simulink model "banc_essai_dec"  (R2021a)
settings: Solver=ode45  StartTime=0.0  StopTime=tfin  FixedStep=0.001  RelTol=1e-09  EnableMultiTasking=on
values from neighbouring files (symbols this model uses):
  A_phi = [A_plaque(1,1),    A_plaque(1,4),  A_plaque(1,7) ... (first row only)    [decouplage.m]
  A_teta = [A_plaque(2,2),    A_plaque(2,5),  A_plaque(2,8) ... (first row only)    [decouplage.m]
  A_x = [A_sphere(1,1), A_sphere(1,3) ... (first row only)    [decouplage.m]
  A_y = [A_sphere(2,2), A_sphere(2,4) ... (first row only)    [decouplage.m]
  A_z = [A_plaque(3,3),    A_plaque(3,6),  A_plaque(3,9) ... (first row only)    [decouplage.m]
  B_phi = [            0 ... (first row only)    [decouplage.m]
  B_teta = [             0 ... (first row only)    [decouplage.m]
  B_x = [            0 ... (first row only)    [decouplage.m]
  B_y = [             0 ... (first row only)    [decouplage.m]
  B_z = [             0 ... (first row only)    [decouplage.m]
  C_phi = [C_plaque(1,1), 0,  0]    [decouplage.m]
  C_teta = [C_plaque(1,1), 0,  0]    [decouplage.m]
  C_x = [C_sphere(1,1), C_sphere(1,3) ... (first row only)    [decouplage.m]
  C_y = [C_sphere(2,2), C_sphere(2,4) ... (first row only)    [decouplage.m]
  C_z = [C_plaque(1,1), 0,  0]    [decouplage.m]
  D_phi = [0]    [decouplage.m]
  D_teta = [0]    [decouplage.m]
  D_x = [ 0;  0]    [decouplage.m]
  D_y = [ 0;  0]    [decouplage.m]
  D_z = [0]    [decouplage.m]
  z_eq = .015    (= 0.015)    [decouplage.m]
undefined symbols (not defined in the file or in its folder): V_eq, Vmax, XA, XB, XC, YB, YC
settings Model: Creator=delafontaine  LastModifiedBy=User
settings SolverCC: AlgebraicLoopSolver=LineSearch
settings DataIOCC: LimitDataPoints=on  SaveFormat=Array  SignalLoggingSaveFormat=ModelDataLogs  ReturnWorkspaceOutputs=off
settings OptimizationCC: LifeSpan=inf
settings DebuggingCC: UnderspecifiedInitializationDetection=Classic  MergeDetectMultiDrivingBlocksExec=none  MultiTaskDSMMsg=warning  MultiTaskCondExecSysMsg=none  SFUnexpectedBacktrackingDiag=warning  SFNoUnconditionalDefaultTransitionDiag=warning  SFExecutionAtInitializationDiag=none  SFMachineParentedDataDiag=warning  ArithmeticOperatorsInVariantConditions=warning
settings HardwareCC: ProdBitPerPointer=32  ProdBitPerSizeT=32  ProdBitPerPtrDiffT=32  ProdLargestAtomicFloat=None  ProdIntDivRoundTo=Undefined  ProdEndianess=Unspecified  ProdWordSize=32  ProdHWDeviceType=32-bit Generic
settings ModelReferenceCC: PropagateSignalLabelsOutOfModel=off
settings SFSimCC: SimUseLocalCustomCode=off  CustomCodeUndefinedFunction=UseInterfaceOnly
settings RTWCC: RTWUseLocalCustomCode=off
settings CodeAppCC: StateflowObjectComments=on
settings GRTTargetCC: TargetLangStandard=C89/C90 (ANSI)
settings ConfigComp: CovMetricSettings=dw  CovSaveCumulativeToWorkspaceVar=on  CovSaveSingleToWorkspaceVar=on  CovExternalEMLEnable=off  CovSFcnEnable=off

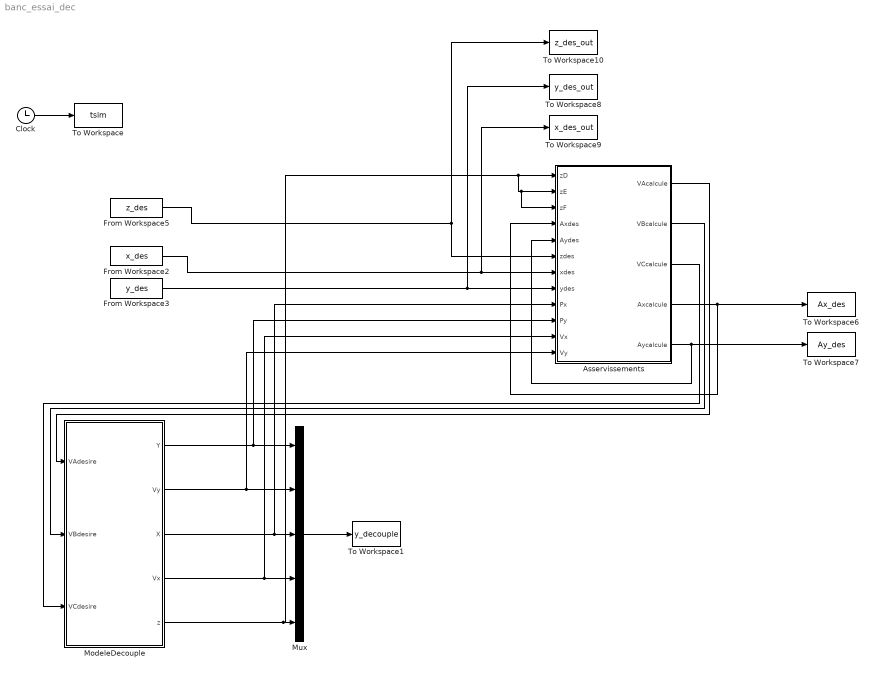
== system banc_essai_dec ==
  Asservissements : Subsystem
      mask help: Simulink:masks:GenSFuncDesc_MD
      mask Help: eval('feval(''rtwprivate'',''rtwhelpview'',''rtw_sfcn_block'')');
  Clock : Clock
  From Workspace2 : FromWorkspace  VariableName=x_des  Interpolate=off  OutputAfterFinalValue=Holding final value
  From Workspace3 : FromWorkspace  VariableName=y_des  Interpolate=off  OutputAfterFinalValue=Holding final value
  From Workspace5 : FromWorkspace  VariableName=z_des  Interpolate=off  OutputAfterFinalValue=Holding final value
  ModeleDecouple : Subsystem
      mask help: Simulink:masks:GenSFuncDesc_MD
      mask Help: eval('feval(''rtwprivate'',''rtwhelpview'',''rtw_sfcn_block'')');
  Mux : Mux  Inputs=5
  To Workspace : ToWorkspace  VariableName=tsim  SampleTime=-1
  To Workspace1 : ToWorkspace  VariableName=y_decouple  SampleTime=-1
  To Workspace10 : ToWorkspace  VariableName=z_des_out  SampleTime=-1
  To Workspace6 : ToWorkspace  VariableName=Ax_des  SampleTime=-1
  To Workspace7 : ToWorkspace  VariableName=Ay_des  SampleTime=-1
  To Workspace8 : ToWorkspace  VariableName=y_des_out  SampleTime=-1
  To Workspace9 : ToWorkspace  VariableName=x_des_out  SampleTime=-1
  wires:
  Mux/1 -> To Workspace1/1
  Clock/1 -> To Workspace/1
  From Workspace5/1 -> Asservissements/6(zdes), To Workspace10/1
  From Workspace3/1 -> Asservissements/8(ydes), To Workspace8/1
  From Workspace2/1 -> Asservissements/7(xdes), To Workspace9/1
  Asservissements/4(Axcalcule) -> Asservissements/4(Axdes), To Workspace6/1
  Asservissements/5(Aycalcule) -> Asservissements/5(Aydes), To Workspace7/1
  Asservissements/1(VAcalcule) -> ModeleDecouple/1(VAdesire)
  Asservissements/2(VBcalcule) -> ModeleDecouple/2(VBdesire)
  Asservissements/3(VCcalcule) -> ModeleDecouple/3(VCdesire)
  ModeleDecouple/1(Y) -> Asservissements/10(Py), Mux/1
  ModeleDecouple/2(Vy) -> Asservissements/12(Vy), Mux/2
  ModeleDecouple/3(X) -> Asservissements/9(Px), Mux/3
  ModeleDecouple/4(Vx) -> Asservissements/11(Vx), Mux/4
  ModeleDecouple/5(z) -> Asservissements/3(zF), Asservissements/2(zE), Asservissements/1(zD), Mux/5

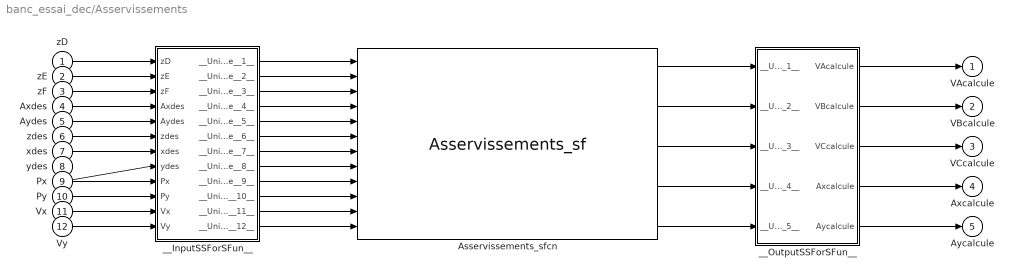
== system banc_essai_dec/Asservissements ==
  zD : Inport
  zE : Inport  Port=2
  zF : Inport  Port=3
  Axdes : Inport  Port=4
  Aydes : Inport  Port=5
  zdes : Inport  Port=6
  xdes : Inport  Port=7
  ydes : Inport  Port=8
  Px : Inport  Port=9
  Py : Inport  Port=10
  Vx : Inport  Port=11
  Vy : Inport  Port=12
  Asservissements_sfcn : S-Function  FunctionName=Asservissements_sf  SFunctionModules=""  SFunctionDeploymentMode=off  EnableBusSupport=off  mask{rtw_sf_name=Asservissements_sf, showVar=off}
      mask prompts: rtw_sf_name "Simulink:masks:GenSFuncName_MP"; showVar "Simulink:masks:GenSFuncShowModuleList_MP"
      mask help: Simulink:masks:GenSFuncDesc_MD
      mask init:
      | displist = '';
      | if ~strcmp(get_param(gcb, 'FunctionName'), rtw_sf_name);
      |   set_param(gcb, 'FunctionName', rtw_sf_name);
      | end
      | % Check if we are generating code
      | rtw_mode = false;
      | if strcmpi(get_param(bdroot(gcb),'SimulationStatus'),'Initializing')
      | 	rtw_mode = strcmpi(get_param(bdroot(gcb),'BuildingRTWCode'),'on') && ...
      | 		~strcmpi(get_param(bdroot(gcb),'TargetStyle'),'SimulationTarget');
      | end
      | if showVar || rtw_mode
      | 	if exist('rtwsfunc') == 2 | exist('rtwsfunc') == 6
      | 		tmplist = rtwsfunc(rtw_sf_name,gcb);
      | 		tmplist = DAStudio.message('Simulink:masks:GenSFuncListOfModules_IC', tmplist);
      | 	elseif showVar
      | 		tmplist1 = DAStudio.message('Simulink:masks:GenSFuncListOfModules_IC', '');
      |         tmplist2 = DAStudio.message('Simulink:masks:GenSFuncNotLicensed_IC');
      |         tmplist = [tmplist1 tmplist2];
      |  	end
      | end
      | if showVar
      |   displist = tmplist;
      | end
      settings: CopyFcn=|
      | if ~strcmp(get_param(gcb,'Linkstatus'),'none') && ...
      | ~strcmp(get_param(gcb,'Linkstatus'),'implicit')
      |   set_param(gcb,'LinkStatus','none');
      | end
      mask Help: eval('feval(''rtwprivate'',''rtwhelpview'',''rtw_sfcn_block'')');
      mask Display:
      | port_label('input',1,'zD');
      | port_label('input',2,'zE');
      | port_label('input',3,'zF');
      | port_label('input',4,'Axdes');
      | port_label('input',5,'Aydes');
      | port_label('input',6,'zdes');
      | port_label('input',7,'xdes');
      | port_label('input',8,'ydes');
      | port_label('input',9,'Px');
      | port_label('input',10,'Py');
      | port_label('input',11,'Vx');
      | port_label('input',12,'Vy');
      | port_label('output',1,'VAcalcule');
      | port_label('output',2,'VBcalcule');
      | port_label('output',3,'VCcalcule');
      | port_label('output',4,'Axcalcule');
      | port_label('output',5,'Aycalcule');
  __InputSSForSFun__ : Subsystem
  __OutputSSForSFun__ : Subsystem
  VAcalcule : Outport
  VBcalcule : Outport  Port=2
  VCcalcule : Outport  Port=3
  Axcalcule : Outport  Port=4
  Aycalcule : Outport  Port=5
  wires:
  zD/1 -> __InputSSForSFun__/1(zD)
  zE/1 -> __InputSSForSFun__/2(zE)
  zF/1 -> __InputSSForSFun__/3(zF)
  Axdes/1 -> __InputSSForSFun__/4(Axdes)
  Aydes/1 -> __InputSSForSFun__/5(Aydes)
  zdes/1 -> __InputSSForSFun__/6(zdes)
  xdes/1 -> __InputSSForSFun__/7(xdes)
  ydes/1 -> __InputSSForSFun__/8(ydes)
  Px/1 -> __InputSSForSFun__/9(Px)
  Py/1 -> __InputSSForSFun__/10(Py)
  Vx/1 -> __InputSSForSFun__/11(Vx)
  Vy/1 -> __InputSSForSFun__/12(Vy)
  __InputSSForSFun__/1(__UniqueOutportName__1__) -> Asservissements_sfcn/1
  __InputSSForSFun__/2(__UniqueOutportName__2__) -> Asservissements_sfcn/2
  __InputSSForSFun__/3(__UniqueOutportName__3__) -> Asservissements_sfcn/3
  __InputSSForSFun__/4(__UniqueOutportName__4__) -> Asservissements_sfcn/4
  __InputSSForSFun__/5(__UniqueOutportName__5__) -> Asservissements_sfcn/5
  __InputSSForSFun__/6(__UniqueOutportName__6__) -> Asservissements_sfcn/6
  __InputSSForSFun__/7(__UniqueOutportName__7__) -> Asservissements_sfcn/7
  __InputSSForSFun__/8(__UniqueOutportName__8__) -> Asservissements_sfcn/8
  __InputSSForSFun__/9(__UniqueOutportName__9__) -> Asservissements_sfcn/9
  __InputSSForSFun__/10(__UniqueOutportName__10__) -> Asservissements_sfcn/10
  __InputSSForSFun__/11(__UniqueOutportName__11__) -> Asservissements_sfcn/11
  __InputSSForSFun__/12(__UniqueOutportName__12__) -> Asservissements_sfcn/12
  Asservissements_sfcn/1 -> __OutputSSForSFun__/1(__UniqueInportName__1__)
  Asservissements_sfcn/2 -> __OutputSSForSFun__/2(__UniqueInportName__2__)
  Asservissements_sfcn/3 -> __OutputSSForSFun__/3(__UniqueInportName__3__)
  Asservissements_sfcn/4 -> __OutputSSForSFun__/4(__UniqueInportName__4__)
  Asservissements_sfcn/5 -> __OutputSSForSFun__/5(__UniqueInportName__5__)
  __OutputSSForSFun__/1(VAcalcule) -> VAcalcule/1
  __OutputSSForSFun__/2(VBcalcule) -> VBcalcule/1
  __OutputSSForSFun__/3(VCcalcule) -> VCcalcule/1
  __OutputSSForSFun__/4(Axcalcule) -> Axcalcule/1
  __OutputSSForSFun__/5(Aycalcule) -> Aycalcule/1

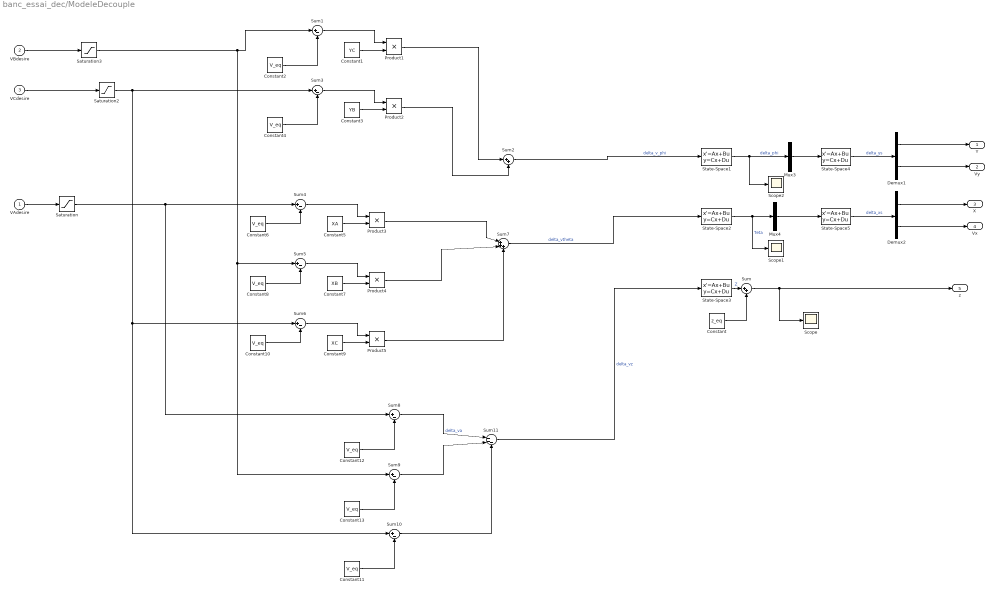
== system banc_essai_dec/ModeleDecouple ==
  VAdesire : Inport
  VBdesire : Inport  Port=2
  VCdesire : Inport  Port=3
  Constant : Constant  Value=z_eq
  Constant1 : Constant  Value=YC
  Constant{2,4,6,8,10..13} (8 alike) : Constant  Value=V_eq
  Constant3 : Constant  Value=YB
  Constant5 : Constant  Value=XA
  Constant7 : Constant  Value=XB
  Constant9 : Constant  Value=XC
  Demux1 : Demux  Outputs=2
  Demux2 : Demux  Outputs=2
  Mux3 : Mux  Inputs=1
  Mux4 : Mux  Inputs=1
  Product{1..5} (5 alike) : Product
  Saturation : Saturate  UpperLimit=0  LowerLimit=-Vmax
  Saturation2 : Saturate  UpperLimit=0  LowerLimit=-Vmax
  Saturation3 : Saturate  UpperLimit=0  LowerLimit=-Vmax
  Scope : Scope
  Scope1 : Scope
  Scope2 : Scope
  State-Space1 : StateSpace  A=A_phi  B=B_phi  C=C_phi  D=D_phi  InitialCondition=0  AbsoluteTolerance=1e-10
  State-Space2 : StateSpace  A=A_teta  B=B_teta  C=C_teta  D=D_teta  InitialCondition=0  AbsoluteTolerance=1e-10
  State-Space3 : StateSpace  A=A_z  B=B_z  C=C_z  D=D_z  InitialCondition=0.03  AbsoluteTolerance=1e-10
  State-Space4 : StateSpace  A=A_y  B=B_y  C=C_y  D=D_y  InitialCondition=0  AbsoluteTolerance=1e-10
  State-Space5 : StateSpace  A=A_x  B=B_x  C=C_x  D=D_x  InitialCondition=0  AbsoluteTolerance=1e-10
  Sum : Sum  Inputs=|++
  Sum{1,3..6,8..10} (8 alike) : Sum  Inputs=|+-
  Sum11 : Sum  Inputs=|---
  Sum2 : Sum  Inputs=|++
  Sum7 : Sum  Inputs=|+++
  Y : Outport
  Vy : Outport  Port=2
  X : Outport  Port=3
  Vx : Outport  Port=4
  z : Outport  Port=5
  wires:
  State-Space3/1 -> Sum/1  "Z"
  Sum2/1 -> State-Space1/1  "delta_v_phi"
  Constant/1 -> Sum/2
  State-Space4/1 -> Demux1/1  "delta_ys"
  Mux4/1 -> State-Space5/1
  State-Space5/1 -> Demux2/1  "delta_xs"
  State-Space2/1 -> Scope1/1, Mux4/1  "Teta"
  State-Space1/1 -> Scope2/1, Mux3/1  "delta_phi"
  Mux3/1 -> State-Space4/1
  Constant2/1 -> Sum1/2
  Sum1/1 -> Product1/1
  Constant1/1 -> Product1/2
  Product1/1 -> Sum2/1
  VCdesire/1 -> Saturation2/1
  Sum3/1 -> Product2/1
  Constant4/1 -> Sum3/2
  Constant3/1 -> Product2/2
  Product2/1 -> Sum2/2
  VBdesire/1 -> Saturation3/1
  Constant8/1 -> Sum5/2
  Sum5/1 -> Product4/1
  Constant7/1 -> Product4/2
  VAdesire/1 -> Saturation/1
  Sum4/1 -> Product3/1
  Product3/1 -> Sum7/1
  Product4/1 -> Sum7/2
  Constant5/1 -> Product3/2
  Constant6/1 -> Sum4/2
  Sum6/1 -> Product5/1
  Constant9/1 -> Product5/2
  Constant10/1 -> Sum6/2
  Product5/1 -> Sum7/3
  Sum7/1 -> State-Space2/1  "delta_vtheta"
  Constant13/1 -> Sum9/2
  Constant11/1 -> Sum10/2
  Constant12/1 -> Sum8/2
  Sum8/1 -> Sum11/1  "delta_va"
  Sum9/1 -> Sum11/2
  Sum10/1 -> Sum11/3
  Sum11/1 -> State-Space3/1  "delta_vz"
  Demux1/1 -> Y/1
  Demux1/2 -> Vy/1
  Demux2/1 -> X/1
  Demux2/2 -> Vx/1
  Sum/1 -> Scope/1, z/1
  Saturation/1 -> Sum8/1, Sum4/1
  Saturation2/1 -> Sum3/1, Sum10/1, Sum6/1
  Saturation3/1 -> Sum9/1, Sum5/1, Sum1/1

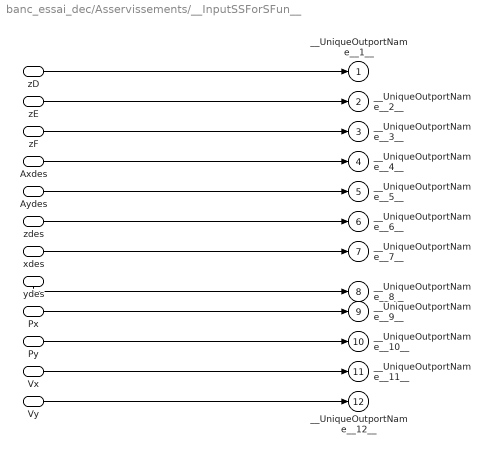
== system banc_essai_dec/Asservissements/__InputSSForSFun__ ==
  zD : Inport
  zE : Inport  Port=2
  zF : Inport  Port=3
  Axdes : Inport  Port=4
  Aydes : Inport  Port=5
  zdes : Inport  Port=6
  xdes : Inport  Port=7
  ydes : Inport  Port=8
  Px : Inport  Port=9
  Py : Inport  Port=10
  Vx : Inport  Port=11
  Vy : Inport  Port=12
  __UniqueOutportName__1__ : Outport
  __UniqueOutportName__2__ : Outport  Port=2
  __UniqueOutportName__3__ : Outport  Port=3
  __UniqueOutportName__4__ : Outport  Port=4
  __UniqueOutportName__5__ : Outport  Port=5
  __UniqueOutportName__6__ : Outport  Port=6
  __UniqueOutportName__7__ : Outport  Port=7
  __UniqueOutportName__8__ : Outport  Port=8
  __UniqueOutportName__9__ : Outport  Port=9
  __UniqueOutportName__10__ : Outport  Port=10
  __UniqueOutportName__11__ : Outport  Port=11
  __UniqueOutportName__12__ : Outport  Port=12
  wires:
  zD/1 -> __UniqueOutportName__1__/1
  zE/1 -> __UniqueOutportName__2__/1
  zF/1 -> __UniqueOutportName__3__/1
  Axdes/1 -> __UniqueOutportName__4__/1
  Aydes/1 -> __UniqueOutportName__5__/1
  zdes/1 -> __UniqueOutportName__6__/1
  xdes/1 -> __UniqueOutportName__7__/1
  ydes/1 -> __UniqueOutportName__8__/1
  Px/1 -> __UniqueOutportName__9__/1
  Py/1 -> __UniqueOutportName__10__/1
  Vx/1 -> __UniqueOutportName__11__/1
  Vy/1 -> __UniqueOutportName__12__/1

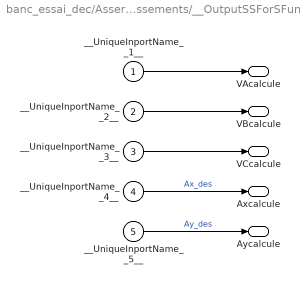
== system banc_essai_dec/Asservissements/__OutputSSForSFun__ ==
  __UniqueInportName__1__ : Inport
  __UniqueInportName__2__ : Inport  Port=2
  __UniqueInportName__3__ : Inport  Port=3
  __UniqueInportName__4__ : Inport  Port=4
  __UniqueInportName__5__ : Inport  Port=5
  VAcalcule : Outport
  VBcalcule : Outport  Port=2
  VCcalcule : Outport  Port=3
  Axcalcule : Outport  Port=4
  Aycalcule : Outport  Port=5
  wires:
  __UniqueInportName__1__/1 -> VAcalcule/1
  __UniqueInportName__2__/1 -> VBcalcule/1
  __UniqueInportName__3__/1 -> VCcalcule/1
  __UniqueInportName__4__/1 -> Axcalcule/1  "Ax_des"
  __UniqueInportName__5__/1 -> Aycalcule/1  "Ay_des"
